simulink model "MATE_HDLsolver_myFirstCircuit"  (R2024b)
settings: Solver=FixedStepDiscrete  StartTime=0.0  StopTime=0.05  FixedStep=Ts  MaxStep=100e-6  RelTol=1e-4
PostLoadFcn:
  | Ts=1e-6; nb_sw=3; nb_lc=2;nb_r=1;nb_src=1; nb_out=3; rL=1.2;rC=100;L=1e-3; C=1e-5; LpejoSw=1e-6;h=Ts; MAX_INPUTS=16;
  | MAX_OUTPUTS=16;
  | MAX_SWITCHES=8;
  | MAX_INPUTS=16;
InitFcn:
  | Ts=1e-6; nb_sw=3; nb_lc=2;nb_r=1;nb_src=1; nb_out=3; rL=1.2;rC=100;L=1e-3; C=1e-5; LpejoSw=1e-6;h=Ts; MAX_INPUTS=16;
  | MAX_OUTPUTS=16;
  | MAX_SWITCHES=8;
  | MAX_INPUTS=16;
undefined symbols (not defined in the file or in its folder): MATE_SOC
libraries: fl_lib x31, nesl_utility x13, simetranss x5, simulink x2, ee_lib x2, eeGeneralControl x2
Description:
  | Copyright 2008-2010 The MathWorks, Inc.
settings Model: ARTEMISmethode_block_infos=$$__separator__$$  Creator=Kyle Diller
settings SolverCC: AlgebraicLoopSolver=TrustRegion
settings DataIOCC: SaveFormat=Array  SignalLoggingSaveFormat=ModelDataLogs  ReturnWorkspaceOutputs=off  SignalLoggingName=sigsOut
settings OptimizationCC: BlockReduction=off  BooleanDataType=off  ConditionallyExecuteInputs=off  OptimizeBlockIOStorage=off  BufferReuse=off  GlobalBufferReuse=off  ExpressionFolding=off  ExpressionDepthLimit=2147483647  LocalBlockOutputs=off  InitFltsAndDblsToZero=on  LifeSpan=inf
settings DebuggingCC: SaveWithParameterizedLinksMsg=none  UnderspecifiedInitializationDetection=Classic  MergeDetectMultiDrivingBlocksExec=none  CheckExecutionContextPreStartOutputMsg=on  SignalResolutionControl=TryResolveAllWithWarning  MultiTaskDSMMsg=warning  MultiTaskCondExecSysMsg=none  SigSpecEnsureSampleTimeMsg=none  FcnCallInpInsideContextMsg=warning  UnconnectedInputMsg=warning  UnconnectedOutputMsg=warning  UnconnectedLineMsg=warning  AllowSymbolicDim=off  StateNameClashWarn=warning  SFUnexpectedBacktrackingDiag=warning  SFNoUnconditionalDefaultTransitionDiag=warning  SFExecutionAtInitializationDiag=none  ArithmeticOperatorsInVariantConditions=warning
settings HardwareCC: ProdBitPerPointer=32  ProdBitPerSizeT=32  ProdBitPerPtrDiffT=32  ProdLargestAtomicFloat=None  ProdIntDivRoundTo=Undefined  ProdEndianess=Unspecified  ProdWordSize=32  ProdHWDeviceType=Specified  TargetUnknown=on
settings ModelReferenceCC: EnableRefExpFcnMdlSchedulingChecks=on  PropagateSignalLabelsOutOfModel=off
settings SFSimCC: SimUseLocalCustomCode=off  CustomCodeUndefinedFunction=UseInterfaceOnly
settings RTWCC: RTWUseLocalCustomCode=off  GPUComputeCapability=3.5
settings CodeAppCC: StateflowObjectComments=on
settings GRTTargetCC: TargetFcnLib=ansi_tfl_tmw.mat  TargetLangStandard=C89/C90 (ANSI)  CombineOutputUpdateFcns=off  GRTInterface=on
settings ConfigComp: CovMetricSettings=dw  CovSaveCumulativeToWorkspaceVar=on  CovSaveSingleToWorkspaceVar=on  CovExternalEMLEnable=off
settings SimscapeCC: SimscapeNormalizeSystem=off

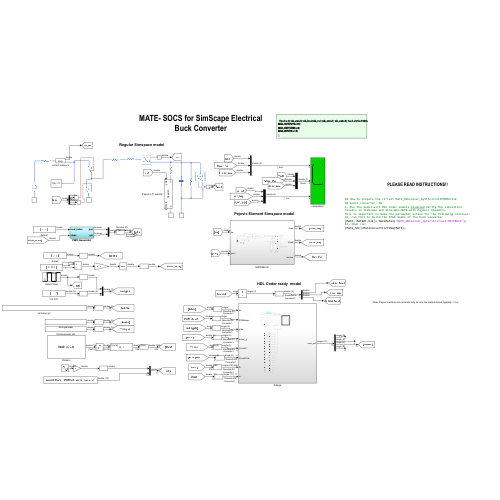
[thumbnail: Simulink's stored preview of the top-level diagram]
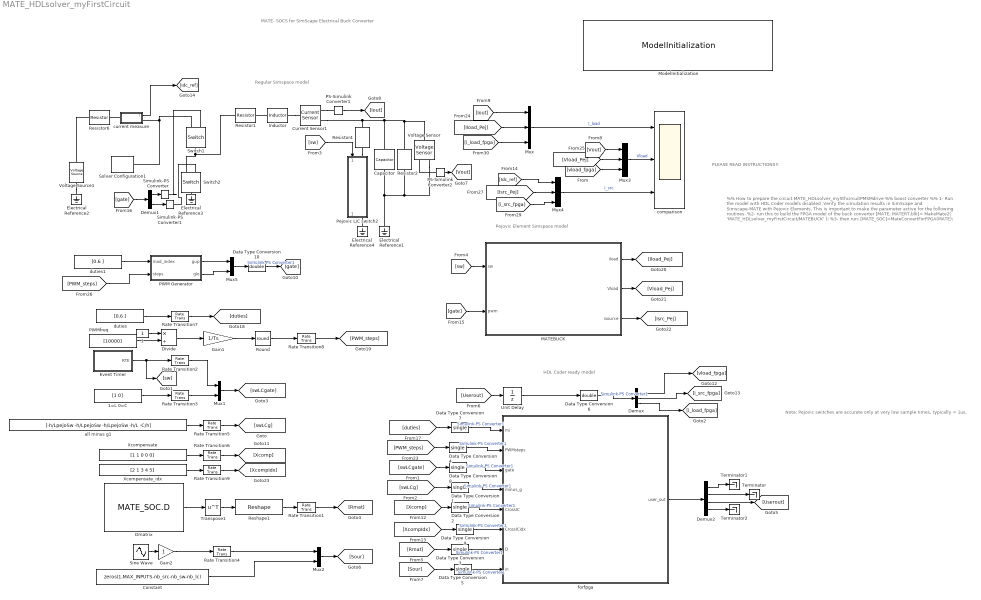
== system MATE_HDLsolver_myFirstCircuit ==
  note: Regular Simspace model
  note: Note: Pejovic switches are accurate only at very low sample times, typically < 1us,
  note: MATE- SOCS for SimScape Electrical
      | Buck Converter
  note: Pejovic Element Simspace model
  note: PLEASE READ INSTRUCTIONS!!
  note: %% How to prepare the circuit MATE_HDLsolver_my5thcircuitPMSMdrive
      | %% boost converter %%
      | 1- Run the model with HDL Coder models disabled .Verify the simulation results in SimScape and Simscape-MATE with Pejovic Elements.
      | This is important to make the parameter active for the following routines.
      | %2- run this to build the FPGA model of the buck converter
      | [MATE, MATERT,blk]= MakeMate2( 'MATE_HDLsolver_myFirstCircuit/MATEBUCK' );
      | %3- then run:
      | [MATE_SOC]=MateConvertForFPGA(MATE);
  note: HDL Coder ready model
  " Event Timer" : Subsystem  Tag=RTEcontrol_s38shd7k88  LoadFcn=|  mask(Timer){is=0 (off), t=[0.01 0.02 0.03 0.04 ], Tmax=0.07, Ts=Ts}
      | xx=get_param(gcb,'linkstatus');      
      | if isequal(xx,'inactive')            
      | set_param(gcb,'linkstatus','restore')
      | end
      mask prompts: is "Initial state"; t "Transition times (s):"; Tmax "Repeat period (s)"; Ts "Sample time (s)"
      mask help: This block generates a Simulink control signal changing at specified transition times.
      mask init:
      | iss=get_param(gcb,'is');
      | if isequal(iss,'0 (off)')
      |     sw(1)=0;
      |     sw(2)=0;
      | else
      |     sw(1)=1;
      |     sw(2)=1;
      | end
      | st(1)=0;
      | st(2)=t(1);
      | 
      | if t(1)==0,
      |    h=errordlg(' The first time specified must be greater than 0 ' , 'Parameter error');
      | end
      | 
      | i=3;
      | tog=0;
      | ptr=2;
      | while length(sw)<=2*length(t)
      |     if tog==0
      |         st=[st st(end)+Ts];
      |         sw=[sw 1-sw(end)];
      |         tog=1;
      |     else
      |         st=[st t(ptr)];
      |         sw=[sw sw(end)];
      |         ptr=ptr+1;
      |         tog=0;
      |     end
      | 
      | end
      |  %st=[st Tmax-Ts Tmax+Ts]
      | % sw=[sw sw(end) sw(1)]
      mask TypeOptions is: 0 (off) | 1 (on)
      mask Display:
      | %plot(0,0,100,100,[70,40,40,20,20,13],[30,30,70,70,30,30]);
      | plot( st(1:end-1), sw(1:end-1) );
  1 : Constant
  1=L 0=C : Constant  Value=[1 0]
  Capacitor : fl_lib/Electrical/Electrical Elements/Capacitor  c=C F  r=0 Ohm  g=0 1/Ohm  i_specify=off  i_priority=None  i=0 A  i_nominal_specify=off  i_nominal_value=1  i_nominal_unit=A  v_specify=off  v_priority=None  v=0 V  v_nominal_specify=off  v_nominal_value=1  v_nominal_unit=V  vc_specify=off  vc_priority=High  vc=0 V  vc_nominal_specify=off  vc_nominal_value=1  vc_nominal_unit=V
  Constant : Constant  Value=zeros(1,MAX_INPUTS-nb_src-nb_sw-nb_lc)
  Current Sensor1 : fl_lib/Electrical/Electrical Sensors/Current Sensor
  Data Type Conversion{1..5,7..9} (8 alike) : DataTypeConversion  OutDataTypeStr=single  RndMeth=Nearest  SaturateOnIntegerOverflow=off
  Data Type Conversion10 : DataTypeConversion  OutDataTypeStr=double  RndMeth=Nearest  SaturateOnIntegerOverflow=off
  Data Type Conversion6 : DataTypeConversion  OutDataTypeStr=double  RndMeth=Nearest  SaturateOnIntegerOverflow=off
  Demux : Demux  Outputs=3
  Demux1 : Demux  Outputs=2
  Demux2 : Demux  Outputs=[nb_sw nb_lc nb_out MAX_OUTPUTS-nb_out-nb_sw-nb_lc]
  Divide : Product  Inputs=*/
  Dmatrix : Constant  Value=MATE_SOC.D
  Electrical Reference{1..4} (4 alike) : fl_lib/Electrical/Electrical Elements/Electrical Reference
  Gain1 : Gain  Gain=1/Ts
  Gain2 : Gain
  Inductor : fl_lib/Electrical/Electrical Elements/Inductor  l=L H  r=0 Ohm  g=1e-9 1/Ohm  i_specify=off  i_priority=None  i=0 A  i_nominal_specify=off  i_nominal_value=1  i_nominal_unit=A  v_specify=off  v_priority=None  v=0 V  v_nominal_specify=off  v_nominal_value=1  v_nominal_unit=V  i_L_specify=off  i_L_priority=High  i_L=0 A  i_L_nominal_specify=off  i_L_nominal_value=1  i_L_nominal_unit=A
  MATEBUCK : Subsystem
  ModelInitialization : simetranss/Usefulls/ModelInitialization  InitFcnX=|  prel=off  posl=on  inif=on  strf=off
      | Ts=1e-6; nb_sw=3; nb_lc=2;nb_r=1;nb_src=1; nb_out=3; rL=1.2;rC=100;L=1e-3; C=1e-5; LpejoSw=1e-6;h=Ts; MAX_INPUTS=16;
      | MAX_OUTPUTS=16;
      | MAX_SWITCHES=8;
      | MAX_INPUTS=16;
  Mux : Mux  Inputs=3
  Mux1 : Mux  Inputs=2
  Mux2 : Mux  Inputs=2
  Mux3 : Mux  Inputs=3
  Mux4 : Mux  Inputs=3
  Mux5 : Mux  Inputs=2
  PS-Simulink Converter1 : nesl_utility/PS-Simulink Converter  PhysicalDomain=network_engine_domain  SubClassName=ps_output  LeftPortType=input  RightPortType=output  PseudoPeriodic=off  Frequencies=[]  VectorFormat=inherit  Unit=inherit  AffineConversion=off
  PS-Simulink Converter2 : nesl_utility/PS-Simulink Converter  PhysicalDomain=network_engine_domain  SubClassName=ps_output  LeftPortType=input  RightPortType=output  PseudoPeriodic=off  Frequencies=[]  VectorFormat=inherit  Unit=inherit  AffineConversion=off
  PWM Generator : Subsystem  Tag=RTEcontrol_s38shd7k88
  PWMfreq : Constant  Value=[10000]
  Pejovic L/C switch2 : Subsystem  AncestorBlock=simetranss/FPGA/Pejovic L//C switch  mask(Pejovic Switch){Lon=LpejoSw, Ts=Ts}
      mask prompts: Lon "Selected equivalent ON inductance (H)"; Ts "Sample Time (s)"
      mask help:
      | Pejovic switch model in SimScape
      |
      | Implements a single phase switch model using the Pejovic constant admittance method.
      | The user only has to select the equivalent ON-state inductance of the model, the corresponding Capacitance is computed internally.
      |
      | In the Pejovic model, Ts/Lon=Coff/Ts (Backward Euler) resulting in a constant admittance for the DAE solver.
      |
      | Input signals;
      |
      | gate: the switch gate value (1 for ON , 0 for OFF)
      mask init:
      | Coff=Ts*Ts/Lon;
      | Rsw=Lon/Ts;
      | 
      | if Ts>2e-6
      |     warndlg(['Sample Time of ' num2str(Ts) ' s. may be somehow large for the Pejovic switch to be accurate. Sample time below 2 us are recommended.'])
      | end
      mask Display: disp(['Pswitch'])
  Rate Transition{1..9} (9 alike) : RateTransition  OutPortSampleTime=1e-06
  Reshape1 : Reshape
  Resistor1 : fl_lib/Electrical/Electrical Elements/Resistor  R=rL Ohm  i_specify=off  i_priority=None  i=0 A  i_nominal_specify=off  i_nominal_value=1  i_nominal_unit=A  v_specify=off  v_priority=None  v=0 V  v_nominal_specify=off  v_nominal_value=1  v_nominal_unit=V
  Resistor2 : fl_lib/Electrical/Electrical Elements/Resistor  R=rC Ohm  i_specify=off  i_priority=None  i=0 A  i_nominal_specify=off  i_nominal_value=1  i_nominal_unit=A  v_specify=off  v_priority=None  v=0 V  v_nominal_specify=off  v_nominal_value=1  v_nominal_unit=V
  Resistor4 : fl_lib/Electrical/Electrical Elements/Resistor  R=rC Ohm  i_specify=off  i_priority=None  i=0 A  i_nominal_specify=off  i_nominal_value=1  i_nominal_unit=A  v_specify=off  v_priority=None  v=0 V  v_nominal_specify=off  v_nominal_value=1  v_nominal_unit=V
  Resistor6 : fl_lib/Electrical/Electrical Elements/Resistor  R=0.01 Ohm  i_specify=off  i_priority=None  i=0 A  i_nominal_specify=off  i_nominal_value=1  i_nominal_unit=A  v_specify=off  v_priority=None  v=0 V  v_nominal_specify=off  v_nominal_value=1  v_nominal_unit=V
  Round : Rounding  Operator=round
  Simulink-PS Converter : nesl_utility/Simulink-PS Converter  PhysicalDomain=network_engine_domain  SubClassName=ps_input  LeftPortType=input  RightPortType=output  PseudoPeriodic=off  Frequencies=[]  NoiseDistribution=none  NoiseParameters=[]  Unit=1  AffineConversion=off  FilteringAndDerivatives=provide  SimscapeFilterOrder=1  InputFilterTimeConstant=0.001  UdotUserProvided=0
  Simulink-PS Converter1 : nesl_utility/Simulink-PS Converter  PhysicalDomain=network_engine_domain  SubClassName=ps_input  LeftPortType=input  RightPortType=output  PseudoPeriodic=off  Frequencies=[]  NoiseDistribution=none  NoiseParameters=[]  Unit=1  AffineConversion=off  FilteringAndDerivatives=provide  SimscapeFilterOrder=1  InputFilterTimeConstant=0.001  UdotUserProvided=0
  Sine Wave : Sin  Amplitude=0  Bias=100  Frequency=0  SampleTime=0
  Solver Configuration1 : nesl_utility/Solver Configuration  PhysicalDomain=network_engine_domain  SubClassName=solver  LeftPortType=input  RightPortType=generic  Tones=[]  Harmonics=[]  SimulateNoise=off  Profile=off  UseLocalSampling=off  EnableSwitchedLinearOptims=on  FrequencyDomain=off  UseCCode=off  RelTol=0.001  AbsTol=0.001  MinStep=1e-09  ToWorkspace=off  RevertToSquareIcSolve=off  NumHomotopyIterations=100  PhasorMode=off  PhasorModeNumHarmonics=1  ConsistencySolver=NEWTON_XTOL_AFTER_FTOL  IndexReductionMethod=DerivativeReplacement  DoDC=off  ResidualTolerance=1e-09  ConsistencyTolSource=GLOBAL  ConsistencyAbsTol=0.001  ConsistencyRelTol=0.001  ConsistencyTolFactor=0.001  UseLocalSolver=on  LocalSolverChoice=NE_BACKWARD_EULER_ADVANCER  ResolveIndetEquations=on  FunctionEvalNumThread=1  LocalSolverSampleTime=Ts  DoFixedCost=on  MaxNonlinIter=1  MaxModeIter=2  ComputeImpulses=off  ImpulseIterations=2  LinearAlgebra=auto  LinearAlgebraNumThread=0  EquationFormulation=NE_TIME_EF  DelaysMemoryBudget=1024  AutomaticFiltering=on  FilteringTimeConstant=0.001  PartitionStorageMethod=AS_NEEDED  PartitionMemoryBudget=1024  PartitionMethod=ROBUST  MultibodyUseLocalSolver=off  MultibodyLocalSolverChoice=ODE1  MultibodyLocalSolverSampleTime=0.001
  Switch1 : fl_lib/Electrical/Electrical Elements/Switch  R_closed=0.001 Ohm  G_open=1e-8 1/Ohm  Threshold=0.5  i_specify=off  i_priority=None  i=0 A  i_nominal_specify=off  i_nominal_value=1  i_nominal_unit=A  v_specify=off  v_priority=None  v=0 V  v_nominal_specify=off  v_nominal_value=1  v_nominal_unit=V
  Switch2 : fl_lib/Electrical/Electrical Elements/Switch  R_closed=0.001 Ohm  G_open=1e-8 1/Ohm  Threshold=0.5  i_specify=off  i_priority=None  i=0 A  i_nominal_specify=off  i_nominal_value=1  i_nominal_unit=A  v_specify=off  v_priority=None  v=0 V  v_nominal_specify=off  v_nominal_value=1  v_nominal_unit=V
  Terminator : Terminator
  Terminator1 : Terminator
  Terminator2 : Terminator
  Transpose1 : Math  Operator=transpose
  Unit Delay : UnitDelay  SampleTime=-1  HasFrameUpgradeWarning=on
  Voltage Sensor : fl_lib/Electrical/Electrical Sensors/Voltage Sensor
  Voltage Source1 : ee_lib/Sources/Voltage Source  dc_voltage=100 V  ac_voltage=0 V  ac_shift=0 rad  ac_frequency=60 Hz  noise_mode=ee.enum.sources.noise.Disabled  PSD=0 V^2/Hz  sample_time=1e-3 s  repeatability=ee.enum.sources.repeatability.NotRepeatable  user_seed=0  auto_seed=1196140742  i_specify=off  i_priority=None  i=0 A  i_nominal_specify=off  i_nominal_value=1  i_nominal_unit=A  v_specify=off  v_priority=None  v=0 V  v_nominal_specify=off  v_nominal_value=1  v_nominal_unit=V
  Xcompensate : Constant  Value=[1 1 0 0 0]
  Xcompensate_idx : Constant  Value=[2 1 3 4 5]
  all minus g1 : Constant  Value=[-h/LpejoSw -h/LpejoSw -h/LpejoSw -h/L -C/h]
  comparison : Scope  NumInputPorts=3
  current measure : Subsystem
      mask Display: disp('amp')
  duties : Constant  Value=[0.6 ]
  duties1 : Constant  Value=[0.6 ]
  forfpga : Subsystem
  wires:
  [sw] -> Pejovic L/C switch2/1(gate)
  Mux/1 -> comparison/1  "I_load"
  Dmatrix/1 -> Transpose1/1
  " Event Timer"/1(RTE) -> [sw], Rate Transition2/1
  Rate Transition2/1 -> Mux1/1
  Sine Wave/1 -> Gain2/1
  Unit Delay/1 -> Data Type Conversion6/1
  1=L 0=C/1 -> Rate Transition3/1
  Rate Transition3/1 -> Mux1/2
  Mux3/1 -> comparison/2  "Vload"
  [Vout] -> Mux3/1
  [sw] -> MATEBUCK/1(sw)
  Mux1/1 -> [swLCgate]
  all minus g1/1 -> Rate Transition5/1
  Rate Transition5/1 -> [swLCg]
  Gain2/1 -> Rate Transition4/1
  Rate Transition1/1 -> [Rmat]
  [Userout] -> Unit Delay/1
  Rate Transition6/1 -> [Xcomp]
  Xcompensate/1 -> Rate Transition6/1
  [swLCgate] -> Data Type Conversion8/1
  [swLCg] -> Data Type Conversion1/1
  [Xcomp] -> Data Type Conversion2/1
  [Rmat] -> Data Type Conversion3/1
  [Sour] -> Data Type Conversion5/1
  Data Type Conversion8/1 -> forfpga/3(gate)  "Simulink-PS Converter1"
  Data Type Conversion1/1 -> forfpga/4(minus_g)  "Simulink-PS Converter1"
  Data Type Conversion2/1 -> forfpga/5(CrossIC)  "Simulink-PS Converter1"
  Data Type Conversion3/1 -> forfpga/7(D)  "Simulink-PS Converter1"
  Data Type Conversion5/1 -> forfpga/8(in)  "Simulink-PS Converter1"
  Demux/1 -> [vload_fpga]
  Demux/2 -> [i_src_fpga]
  [vload_fpga] -> Mux3/3
  Data Type Conversion6/1 -> Demux/1  "Simulink-PS Converter1"
  [gate] -> MATEBUCK/2(pwm)
  Demux1/2 -> Simulink-PS Converter1/1
  Demux1/1 -> Simulink-PS Converter/1
  [gate] -> Demux1/1
  current measure/1(i) -> [Idc_ref]
  duties/1 -> Rate Transition7/1
  Rate Transition7/1 -> [duties]
  Data Type Conversion7/1 -> forfpga/1(mi)  "Simulink-PS Converter1"
  [duties] -> Data Type Conversion7/1
  Mux2/1 -> [Sour]
  Rate Transition4/1 -> Mux2/1
  Constant/1 -> Mux2/2
  Data Type Conversion4/1 -> forfpga/2(PWMsteps)  "Simulink-PS Converter1"
  Rate Transition8/1 -> [PWM_steps]
  Divide/1 -> Gain1/1
  Gain1/1 -> Round/1
  [PWM_steps] -> Data Type Conversion4/1
  forfpga/1(user_out) -> Demux2/1
  Demux2/2 -> Terminator/1
  MATEBUCK/1(iload) -> [Iload_Pej]
  MATEBUCK/2(Vload) -> [Vload_Pej]
  MATEBUCK/3(isource) -> [Isrc_Pej]
  [Iload_Pej] -> Mux/2
  [i_load_fpga] -> Mux/3
  [Vload_Pej] -> Mux3/2
  Mux4/1 -> comparison/3  "I_src"
  [Idc_ref] -> Mux4/1
  [Isrc_Pej] -> Mux4/2
  Demux2/3 -> [Userout]
  Demux2/1 -> Terminator1/1
  Demux2/4 -> Terminator2/1
  PWMfreq/1 -> Divide/2
  1/1 -> Divide/1
  Demux/3 -> [i_load_fpga]
  [i_src_fpga] -> Mux4/3
  Xcompensate_idx/1 -> Rate Transition9/1
  Rate Transition9/1 -> [XcompIdx]
  [XcompIdx] -> Data Type Conversion9/1
  Data Type Conversion9/1 -> forfpga/6(CrossICidx)  "Simulink-PS Converter1"
  Round/1 -> Rate Transition8/1
  duties1/1 -> PWM Generator/1(mod_index)
  [PWM_steps] -> PWM Generator/2(steps)
  PWM Generator/2(glo) -> Mux5/2
  PWM Generator/1(gup) -> Mux5/1
  Mux5/1 -> Data Type Conversion10/1
  Data Type Conversion10/1 -> [gate]  "Simulink-PS Converter1"
  PS-Simulink Converter2/1 -> [Vout]
  PS-Simulink Converter1/1 -> [Iout]
  [Iout] -> Mux/1
  Transpose1/1 -> Reshape1/1
  Reshape1/1 -> Rate Transition1/1
  connections:
  Switch2/RConn2 -- Resistor1/LConn1 -- Switch1/LConn1
  Switch1/RConn2 -- current measure/RConn1 -- Solver Configuration1/RConn1
  Current Sensor1/RConn1 -- PS-Simulink Converter1/LConn1
  Inductor/LConn1 -- Resistor1/RConn1
  Inductor/RConn1 -- Current Sensor1/LConn1
  Current Sensor1/RConn2 -- Resistor4/LConn1 -- Voltage Sensor/LConn1 -- Resistor2/LConn1 -- Capacitor/LConn1
  Voltage Sensor/RConn2 -- Resistor2/RConn1 -- Capacitor/RConn1 -- Electrical Reference1/LConn1
  Voltage Source1/LConn1 -- Resistor6/LConn1
  Voltage Source1/RConn1 -- Electrical Reference2/LConn1
  Simulink-PS Converter1/RConn1 -- Switch2/RConn1
  Simulink-PS Converter/RConn1 -- Switch1/RConn1
  Electrical Reference3/LConn1 -- Switch2/LConn1
  current measure/LConn1 -- Resistor6/RConn1
  Electrical Reference4/LConn1 -- Pejovic L/C switch2/RConn1
  Resistor4/RConn1 -- Pejovic L/C switch2/LConn1
  PS-Simulink Converter2/LConn1 -- Voltage Sensor/RConn1

== system MATE_HDLsolver_myFirstCircuit/ Event Timer ==
  Repeating Sequence : simulink/Sources/Repeating Sequence  rep_seq_t=st  rep_seq_y=sw
  Repeating Sequence1 : simulink/Sources/Repeating Sequence  Commented=on  rep_seq_t="[0    0.2000    0.2001    0.4000    0.4001    0.6000    2.0000]"  rep_seq_y=|
      | [     1     1     0     0     1     1     1
      | ]
  RTE : Outport  VectorParamsAs1DForOutWhenUnconnected=off
  wires:
  Repeating Sequence/1 -> RTE/1

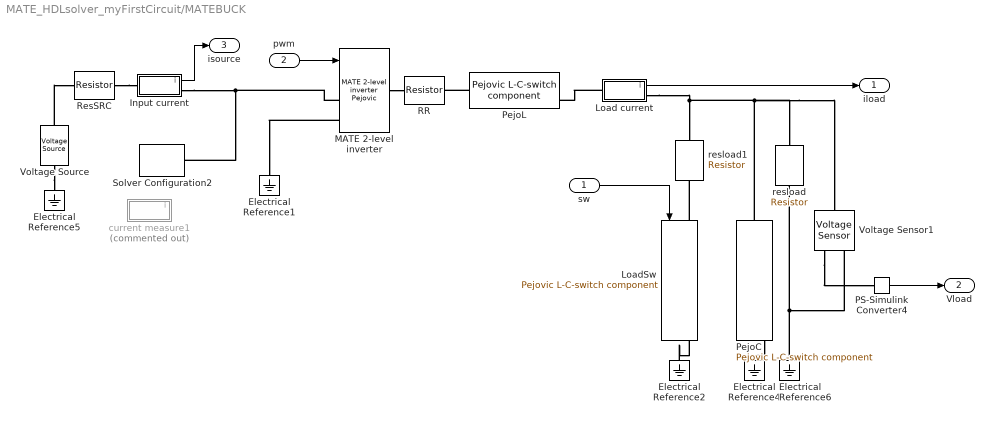
== system MATE_HDLsolver_myFirstCircuit/MATEBUCK ==
  sw : Inport
  pwm : Inport  Port=2
  Electrical Reference{1..2,4..6} (5 alike) : fl_lib/Electrical/Electrical Elements/Electrical Reference
  Input current : Subsystem
  Load current : Subsystem
  LoadSw : simetranss/FPGA/Pejovic L-C-switch component  typ=Switch  Lon=LpejoSw  L=L  C=C  otherSW='coming soon'  Ts=Ts  pcbp=off
  MATE 2-level inverter : simetranss/FPGA/MATE 2-level inverter Pejovic  Lon=1e-6  Ts=Ts
  PS-Simulink Converter4 : nesl_utility/PS-Simulink Converter  PhysicalDomain=network_engine_domain  SubClassName=ps_output  LeftPortType=input  RightPortType=output  PseudoPeriodic=off  Frequencies=[]  VectorFormat=inherit  Unit=inherit  AffineConversion=off
  PejoC : simetranss/FPGA/Pejovic L-C-switch component  typ=Capacitor  Lon=LpejoSw  L=L  C=C  otherSW='coming soon'  Ts=Ts  pcbp=off
  PejoL : simetranss/FPGA/Pejovic L-C-switch component  typ=Inductor  Lon=LpejoSw  L=L  C=C  otherSW='coming soon'  Ts=Ts  pcbp=off
  RR : fl_lib/Electrical/Electrical Elements/Resistor  R=rL Ohm  i_specify=off  i_priority=None  i=0 A  i_nominal_specify=off  i_nominal_value=1  i_nominal_unit=A  v_specify=off  v_priority=None  v=0 V  v_nominal_specify=off  v_nominal_value=1  v_nominal_unit=V
  ResSRC : fl_lib/Electrical/Electrical Elements/Resistor  R=0.01 Ohm  i_specify=off  i_priority=None  i=0 A  i_nominal_specify=off  i_nominal_value=1  i_nominal_unit=A  v_specify=off  v_priority=None  v=0 V  v_nominal_specify=off  v_nominal_value=1  v_nominal_unit=V
  Solver Configuration2 : nesl_utility/Solver Configuration  PhysicalDomain=network_engine_domain  SubClassName=solver  LeftPortType=input  RightPortType=generic  Tones=[]  Harmonics=[]  SimulateNoise=off  Profile=off  UseLocalSampling=off  EnableSwitchedLinearOptims=on  FrequencyDomain=off  UseCCode=off  RelTol=0.001  AbsTol=0.001  MinStep=1e-09  ToWorkspace=off  RevertToSquareIcSolve=off  NumHomotopyIterations=100  PhasorMode=off  PhasorModeNumHarmonics=1  ConsistencySolver=NEWTON_XTOL_AFTER_FTOL  IndexReductionMethod=DerivativeReplacement  DoDC=off  ResidualTolerance=1e-09  ConsistencyTolSource=GLOBAL  ConsistencyAbsTol=0.001  ConsistencyRelTol=0.001  ConsistencyTolFactor=0.001  UseLocalSolver=on  LocalSolverChoice=NE_BACKWARD_EULER_ADVANCER  ResolveIndetEquations=on  FunctionEvalNumThread=1  LocalSolverSampleTime=Ts  DoFixedCost=on  MaxNonlinIter=1  MaxModeIter=2  ComputeImpulses=off  ImpulseIterations=2  LinearAlgebra=auto  LinearAlgebraNumThread=0  EquationFormulation=NE_TIME_EF  DelaysMemoryBudget=1024  AutomaticFiltering=on  FilteringTimeConstant=0.001  PartitionStorageMethod=AS_NEEDED  PartitionMemoryBudget=1024  PartitionMethod=ROBUST  MultibodyUseLocalSolver=off  MultibodyLocalSolverChoice=ODE1  MultibodyLocalSolverSampleTime=0.001
  Voltage Sensor1 : fl_lib/Electrical/Electrical Sensors/Voltage Sensor
  Voltage Source : ee_lib/Sources/Voltage Source  dc_voltage=100 V  ac_voltage=0 V  ac_shift=0 rad  ac_frequency=60 Hz  noise_mode=ee.enum.sources.noise.Disabled  PSD=0 V^2/Hz  sample_time=1e-3 s  repeatability=ee.enum.sources.repeatability.NotRepeatable  user_seed=0  auto_seed=198304613  i_specify=off  i_priority=None  i=0 A  i_nominal_specify=off  i_nominal_value=1  i_nominal_unit=A  v_specify=off  v_priority=None  v=0 V  v_nominal_specify=off  v_nominal_value=1  v_nominal_unit=V
  current measure1 : Subsystem  Commented=on
      mask Display: disp('amp')
  resload : fl_lib/Electrical/Electrical Elements/Resistor  R=rC Ohm  i_specify=off  i_priority=None  i=0 A  i_nominal_specify=off  i_nominal_value=1  i_nominal_unit=A  v_specify=off  v_priority=None  v=0 V  v_nominal_specify=off  v_nominal_value=1  v_nominal_unit=V
  resload1 : fl_lib/Electrical/Electrical Elements/Resistor  R=rC Ohm  i_specify=off  i_priority=None  i=0 A  i_nominal_specify=off  i_nominal_value=1  i_nominal_unit=A  v_specify=off  v_priority=None  v=0 V  v_nominal_specify=off  v_nominal_value=1  v_nominal_unit=V
  iload : Outport
  Vload : Outport  Port=2
  isource : Outport  Port=3
  wires:
  PS-Simulink Converter4/1 -> Vload/1
  sw/1 -> LoadSw/1
  Load current/1(i) -> iload/1
  pwm/1 -> MATE 2-level inverter/1
  Input current/1(i) -> isource/1
  connections:
  Load current/LConn1 -- PejoL/RConn1
  Voltage Source/RConn1 -- Electrical Reference5/LConn1
  Voltage Source/LConn1 -- ResSRC/LConn1
  MATE 2-level inverter/RConn1 -- RR/LConn1
  PejoL/LConn1 -- RR/RConn1
  PejoC/RConn1 -- Electrical Reference4/LConn1
  Voltage Sensor1/RConn1 -- PS-Simulink Converter4/LConn1
  Electrical Reference6/LConn1 -- resload/RConn1 -- Voltage Sensor1/RConn2
  Input current/RConn1 -- MATE 2-level inverter/LConn1 -- Solver Configuration2/RConn1
  Voltage Sensor1/LConn1 -- resload/LConn1 -- Load current/RConn1 -- resload1/LConn1 -- PejoC/LConn1
  MATE 2-level inverter/LConn2 -- Electrical Reference1/LConn1
  LoadSw/LConn1 -- resload1/RConn1
  Electrical Reference2/LConn1 -- LoadSw/RConn1
  ResSRC/RConn1 -- Input current/LConn1

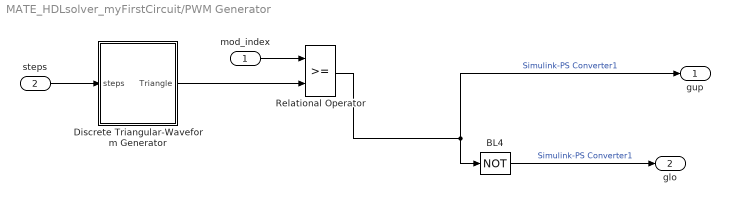
== system MATE_HDLsolver_myFirstCircuit/PWM Generator ==
  mod_index : Inport
  steps : Inport  Port=2
  BL4 : Logic  Operator=NOT  Inputs=1
  Discrete Triangular-Waveform Generator : Subsystem
  Relational Operator : RelationalOperator  OutDataTypeStr=boolean
  gup : Outport  VectorParamsAs1DForOutWhenUnconnected=off
  glo : Outport  Port=2  VectorParamsAs1DForOutWhenUnconnected=off
  wires:
  Discrete Triangular-Waveform Generator/1(Triangle) -> Relational Operator/2
  mod_index/1 -> Relational Operator/1
  steps/1 -> Discrete Triangular-Waveform Generator/1(steps)
  Relational Operator/1 -> gup/1, BL4/1  "Simulink-PS Converter1"
  BL4/1 -> glo/1  "Simulink-PS Converter1"

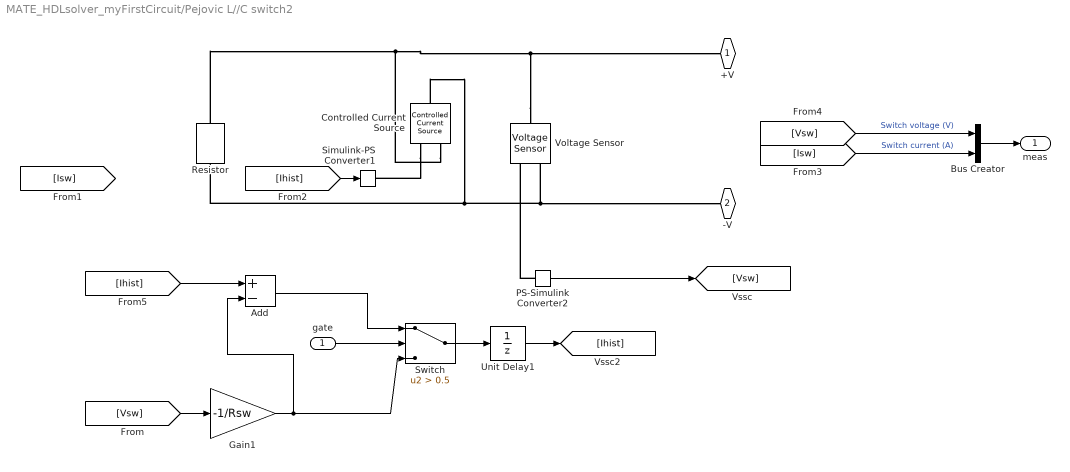
== system MATE_HDLsolver_myFirstCircuit/Pejovic L//C switch2 ==
  gate : Inport
  Add : Sum  Inputs=+-
  Bus Creator : BusCreator  Inputs=2
  Controlled Current Source : fl_lib/Electrical/Electrical Sources/Controlled Current Source
  Gain1 : Gain  Gain=-1/Rsw
  PS-Simulink Converter2 : nesl_utility/PS-Simulink Converter  PhysicalDomain=network_engine_domain  SubClassName=ps_output  LeftPortType=input  RightPortType=output  PseudoPeriodic=off  Frequencies=[]  VectorFormat=inherit  Unit=inherit  AffineConversion=off
  Resistor : fl_lib/Electrical/Electrical Elements/Resistor  R=Rsw Ohm  i_specify=off  i_priority=None  i=0 A  i_nominal_specify=off  i_nominal_value=1  i_nominal_unit=A  v_specify=off  v_priority=None  v=0 V  v_nominal_specify=off  v_nominal_value=1  v_nominal_unit=V
  Simulink-PS Converter1 : nesl_utility/Simulink-PS Converter  PhysicalDomain=network_engine_domain  SubClassName=ps_input  LeftPortType=input  RightPortType=output  PseudoPeriodic=off  Frequencies=[]  NoiseDistribution=none  NoiseParameters=[]  Unit=1  AffineConversion=off  FilteringAndDerivatives=provide  SimscapeFilterOrder=1  InputFilterTimeConstant=0.001  UdotUserProvided=0
  Switch : Switch  Criteria=u2 > Threshold  Threshold=0.5  SaturateOnIntegerOverflow=off  InputSameDT=off
  Unit Delay1 : UnitDelay  SampleTime=-1  HasFrameUpgradeWarning=on
  Voltage Sensor : fl_lib/Electrical/Electrical Sensors/Voltage Sensor
  +V : PMIOPort  Side=Left
  -V : PMIOPort  Port=2  Side=Right
  meas : Outport
  wires:
  Unit Delay1/1 -> [Ihist]
  Add/1 -> Switch/1
  Gain1/1 -> Add/2, Switch/3
  [Ihist] -> Add/1
  PS-Simulink Converter2/1 -> [Vsw]
  gate/1 -> Switch/2
  [Vsw] -> Gain1/1
  Switch/1 -> Unit Delay1/1
  [Ihist] -> Simulink-PS Converter1/1
  [Isw] -> Bus Creator/2  "Switch current (A)"
  [Vsw] -> Bus Creator/1  "Switch voltage (V)"
  Bus Creator/1 -> meas/1
  connections:
  Resistor/RConn1 -- Controlled Current Source/LConn1 -- Voltage Sensor/RConn2 -- -V/RConn1
  PS-Simulink Converter2/LConn1 -- Voltage Sensor/RConn1
  Controlled Current Source/RConn1 -- Simulink-PS Converter1/RConn1
  Voltage Sensor/LConn1 -- +V/RConn1 -- Controlled Current Source/RConn2 -- Resistor/LConn1

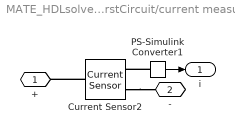
== system MATE_HDLsolver_myFirstCircuit/current measure ==
  Current Sensor2 : fl_lib/Electrical/Electrical Sensors/Current Sensor
  PS-Simulink Converter1 : nesl_utility/PS-Simulink Converter  PhysicalDomain=network_engine_domain  SubClassName=ps_output  LeftPortType=input  RightPortType=output  PseudoPeriodic=off  Frequencies=[]  VectorFormat=inherit  Unit=inherit  AffineConversion=off
  + : PMIOPort  Side=Left
  - : PMIOPort  Port=2  Side=Right
  i : Outport
  wires:
  PS-Simulink Converter1/1 -> i/1
  connections:
  PS-Simulink Converter1/LConn1 -- Current Sensor2/RConn1
  Current Sensor2/LConn1 -- +/RConn1
  Current Sensor2/RConn2 -- -/RConn1

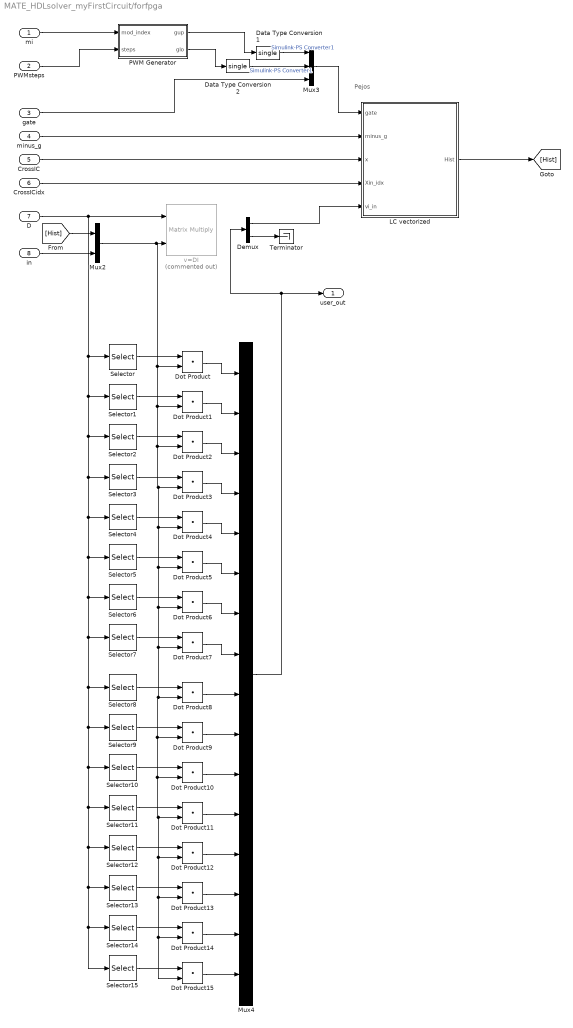
== system MATE_HDLsolver_myFirstCircuit/forfpga ==
  note: Pejos
  mi : Inport
  PWMsteps : Inport  Port=2
  gate : Inport  Port=3
  minus_g : Inport  Port=4
  CrossIC : Inport  Port=5
  CrossICidx : Inport  Port=6
  D : Inport  Port=7
  in : Inport  Port=8
  Data Type Conversion1 : DataTypeConversion  OutDataTypeStr=single  RndMeth=Nearest  SaturateOnIntegerOverflow=off
  Data Type Conversion2 : DataTypeConversion  OutDataTypeStr=single  RndMeth=Nearest  SaturateOnIntegerOverflow=off
  Demux : Demux  Outputs=[nb_sw+nb_lc -1]
  Dot Product{,1..15} (16 alike) : DotProduct  OutDataTypeStr=Inherit: Inherit via internal rule
  LC vectorized : Subsystem
  Mux2 : Mux  Inputs=2
  Mux3 : Mux  Inputs=3
  Mux4 : Mux  Inputs=16
  PWM Generator : Subsystem  Tag=RTEcontrol_s38shd7k88
  Selector : Selector  InputPortWidth=16*16  IndexOptions=Index vector (dialog)  Indices=[1:16]  OutputSizes=1
  Selector1 : Selector  InputPortWidth=16*16  IndexOptions=Index vector (dialog)  Indices=[1:16]+16*1  OutputSizes=1
  Selector10 : Selector  InputPortWidth=16*16  IndexOptions=Index vector (dialog)  Indices=[1:16]+16*10  OutputSizes=1
  Selector11 : Selector  InputPortWidth=16*16  IndexOptions=Index vector (dialog)  Indices=[1:16]+16*11  OutputSizes=1
  Selector12 : Selector  InputPortWidth=16*16  IndexOptions=Index vector (dialog)  Indices=[1:16]+16*12  OutputSizes=1
  Selector13 : Selector  InputPortWidth=16*16  IndexOptions=Index vector (dialog)  Indices=[1:16]+16*13  OutputSizes=1
  Selector14 : Selector  InputPortWidth=16*16  IndexOptions=Index vector (dialog)  Indices=[1:16]+16*14  OutputSizes=1
  Selector15 : Selector  InputPortWidth=16*16  IndexOptions=Index vector (dialog)  Indices=[1:16]+16*15  OutputSizes=1
  Selector2 : Selector  InputPortWidth=16*16  IndexOptions=Index vector (dialog)  Indices=[1:16]+16*2  OutputSizes=1
  Selector3 : Selector  InputPortWidth=16*16  IndexOptions=Index vector (dialog)  Indices=[1:16]+16*3  OutputSizes=1
  Selector4 : Selector  InputPortWidth=16*16  IndexOptions=Index vector (dialog)  Indices=[1:16]+16*4  OutputSizes=1
  Selector5 : Selector  InputPortWidth=16*16  IndexOptions=Index vector (dialog)  Indices=[1:16]+16*5  OutputSizes=1
  Selector6 : Selector  InputPortWidth=16*16  IndexOptions=Index vector (dialog)  Indices=[1:16]+16*6  OutputSizes=1
  Selector7 : Selector  InputPortWidth=16*16  IndexOptions=Index vector (dialog)  Indices=[1:16]+16*7  OutputSizes=1
  Selector8 : Selector  InputPortWidth=16*16  IndexOptions=Index vector (dialog)  Indices=[1:16]+16*8  OutputSizes=1
  Selector9 : Selector  InputPortWidth=16*16  IndexOptions=Index vector (dialog)  Indices=[1:16]+16*9  OutputSizes=1
  Terminator : Terminator
  v=DI : Product  Commented=on  Multiplication=Matrix(*)
  user_out : Outport
  wires:
  in/1 -> Mux2/2
  LC vectorized/1(Hist) -> [Hist]
  minus_g/1 -> LC vectorized/2(minus_g)
  CrossIC/1 -> LC vectorized/3(x)
  Demux/1 -> LC vectorized/5(vi_in)
  mi/1 -> PWM Generator/1(mod_index)
  PWM Generator/1(gup) -> Data Type Conversion1/1
  Mux3/1 -> LC vectorized/1(gate)
  PWMsteps/1 -> PWM Generator/2(steps)
  gate/1 -> Mux3/3
  PWM Generator/2(glo) -> Data Type Conversion2/1
  Demux/2 -> Terminator/1
  [Hist] -> Mux2/1
  Data Type Conversion1/1 -> Mux3/1  "Simulink-PS Converter1"
  Data Type Conversion2/1 -> Mux3/2  "Simulink-PS Converter1"
  CrossICidx/1 -> LC vectorized/4(Xin_idx)
  Selector7/1 -> Dot Product7/1
  Dot Product10/1 -> Mux4/11
  Dot Product9/1 -> Mux4/10
  Dot Product13/1 -> Mux4/14
  Dot Product8/1 -> Mux4/9
  Dot Product11/1 -> Mux4/12
  Dot Product15/1 -> Mux4/16
  Dot Product6/1 -> Mux4/7
  Dot Product/1 -> Mux4/1
  Selector3/1 -> Dot Product3/1
  Dot Product5/1 -> Mux4/6
  Selector2/1 -> Dot Product2/1
  Dot Product1/1 -> Mux4/2
  Dot Product2/1 -> Mux4/3
  Mux4/1 -> Demux/1, user_out/1
  Dot Product7/1 -> Mux4/8
  Selector8/1 -> Dot Product8/1
  Selector10/1 -> Dot Product10/1
  Selector15/1 -> Dot Product15/1
  Selector12/1 -> Dot Product12/1
  Selector11/1 -> Dot Product11/1
  Dot Product12/1 -> Mux4/13
  Selector13/1 -> Dot Product13/1
  Selector4/1 -> Dot Product4/1
  Selector/1 -> Dot Product/1
  Selector6/1 -> Dot Product6/1
  Selector9/1 -> Dot Product9/1
  D/1 -> v=DI/1, Selector1/1, Selector2/1, Selector3/1, Selector4/1, Selector5/1, Selector8/1, Selector14/1, Selector15/1, Selector13/1, Selector12/1, Selector11/1, Selector10/1, Selector9/1, Selector7/1, Selector6/1, Selector/1
  Dot Product14/1 -> Mux4/15
  Selector14/1 -> Dot Product14/1
  Selector1/1 -> Dot Product1/1
  Mux2/1 -> Dot Product9/2, Dot Product10/2, Dot Product11/2, Dot Product12/2, Dot Product13/2, Dot Product14/2, Dot Product15/2, Dot Product8/2, Dot Product7/2, Dot Product6/2, Dot Product5/2, Dot Product4/2, Dot Product3/2, Dot Product2/2, Dot Product1/2, Dot Product/2, v=DI/2
  Dot Product3/1 -> Mux4/4
  Selector5/1 -> Dot Product5/1
  Dot Product4/1 -> Mux4/5

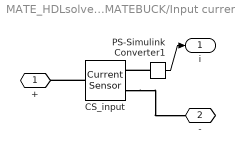
== system MATE_HDLsolver_myFirstCircuit/MATEBUCK/Input current ==
  CS_input : fl_lib/Electrical/Electrical Sensors/Current Sensor
  PS-Simulink Converter1 : nesl_utility/PS-Simulink Converter  PhysicalDomain=network_engine_domain  SubClassName=ps_output  LeftPortType=input  RightPortType=output  PseudoPeriodic=off  Frequencies=[]  VectorFormat=inherit  Unit=inherit  AffineConversion=off
  + : PMIOPort  Side=Left
  - : PMIOPort  Port=2  Side=Right
  i : Outport
  wires:
  PS-Simulink Converter1/1 -> i/1
  connections:
  PS-Simulink Converter1/LConn1 -- CS_input/RConn1
  CS_input/LConn1 -- +/RConn1
  CS_input/RConn2 -- -/RConn1

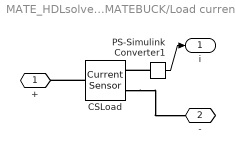
== system MATE_HDLsolver_myFirstCircuit/MATEBUCK/Load current ==
  CSLoad : fl_lib/Electrical/Electrical Sensors/Current Sensor
  PS-Simulink Converter1 : nesl_utility/PS-Simulink Converter  PhysicalDomain=network_engine_domain  SubClassName=ps_output  LeftPortType=input  RightPortType=output  PseudoPeriodic=off  Frequencies=[]  VectorFormat=inherit  Unit=inherit  AffineConversion=off
  + : PMIOPort  Side=Left
  - : PMIOPort  Port=2  Side=Right
  i : Outport
  wires:
  PS-Simulink Converter1/1 -> i/1
  connections:
  CSLoad/RConn2 -- -/RConn1
  CSLoad/LConn1 -- +/RConn1
  PS-Simulink Converter1/LConn1 -- CSLoad/RConn1

== system MATE_HDLsolver_myFirstCircuit/MATEBUCK/current measure1 ==
  Current Sensor2 : fl_lib/Electrical/Electrical Sensors/Current Sensor
  PS-Simulink Converter1 : nesl_utility/PS-Simulink Converter  PhysicalDomain=network_engine_domain  SubClassName=ps_output  LeftPortType=input  RightPortType=output  PseudoPeriodic=off  Frequencies=[]  VectorFormat=inherit  Unit=inherit  AffineConversion=off
  + : PMIOPort  Side=Left
  - : PMIOPort  Port=2  Side=Right
  i : Outport
  wires:
  PS-Simulink Converter1/1 -> i/1
  connections:
  Current Sensor2/RConn2 -- -/RConn1
  Current Sensor2/LConn1 -- +/RConn1
  PS-Simulink Converter1/LConn1 -- Current Sensor2/RConn1

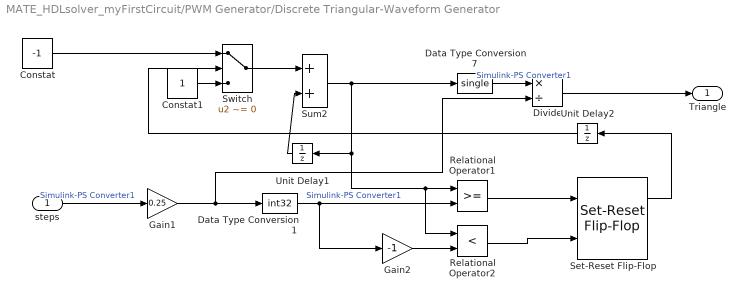
== system MATE_HDLsolver_myFirstCircuit/PWM Generator/Discrete Triangular-Waveform Generator ==
  steps : Inport
  Constat : Constant  Value=-1  OutDataTypeStr=int32
  Constat1 : Constant  OutDataTypeStr=int32
  Data Type Conversion1 : DataTypeConversion  OutDataTypeStr=int32  RndMeth=Nearest  SaturateOnIntegerOverflow=off
  Data Type Conversion7 : DataTypeConversion  OutDataTypeStr=single  RndMeth=Nearest  SaturateOnIntegerOverflow=off
  Divide : Product  Inputs=*/
  Gain1 : Gain  Gain=0.25  SaturateOnIntegerOverflow=on  OutDataTypeStr=Inherit: Same as input  ParamDataTypeStr=Inherit: Same as input
  Gain2 : Gain  Gain=-1  SaturateOnIntegerOverflow=on  OutDataTypeStr=Inherit: Same as input  ParamDataTypeStr=Inherit: Same as input
  Relational Operator1 : RelationalOperator
  Relational Operator2 : RelationalOperator  Operator=<
  Set-Reset Flip-Flop : eeGeneralControl/Set-Reset Flip-Flop  LabelModeActiveChoice=Discrete  UndefState=Set  Q0=0  Ts=Ts
      settings: LibrarySourceBlock=ee_sl_lib/General Control/Set-Reset Flip-Flop
  Sum2 : Sum  InputSameDT=on  SaturateOnIntegerOverflow=on  OutDataTypeStr=Inherit: Same as first input
  Switch : Switch  Criteria=u2 ~= 0
  Unit Delay1 : UnitDelay  SampleTime=Ts  HasFrameUpgradeWarning=on
  Unit Delay2 : UnitDelay  SampleTime=Ts  HasFrameUpgradeWarning=on
  Triangle : Outport  InitialOutput=0  VectorParamsAs1DForOutWhenUnconnected=off
  wires:
  Constat/1 -> Switch/1
  Constat1/1 -> Switch/3
  Switch/1 -> Sum2/1
  Unit Delay1/1 -> Sum2/2
  Sum2/1 -> Relational Operator2/1, Relational Operator1/1, Unit Delay1/1, Data Type Conversion7/1
  Gain1/1 -> Divide/2, Data Type Conversion1/1
  Relational Operator1/1 -> Set-Reset Flip-Flop/1
  Gain2/1 -> Relational Operator2/2
  Relational Operator2/1 -> Set-Reset Flip-Flop/2
  Set-Reset Flip-Flop/1 -> Unit Delay2/1
  Unit Delay2/1 -> Switch/2
  Divide/1 -> Triangle/1
  Data Type Conversion7/1 -> Divide/1  "Simulink-PS Converter1"
  steps/1 -> Gain1/1  "Simulink-PS Converter1"
  Data Type Conversion1/1 -> Gain2/1, Relational Operator1/2  "Simulink-PS Converter1"

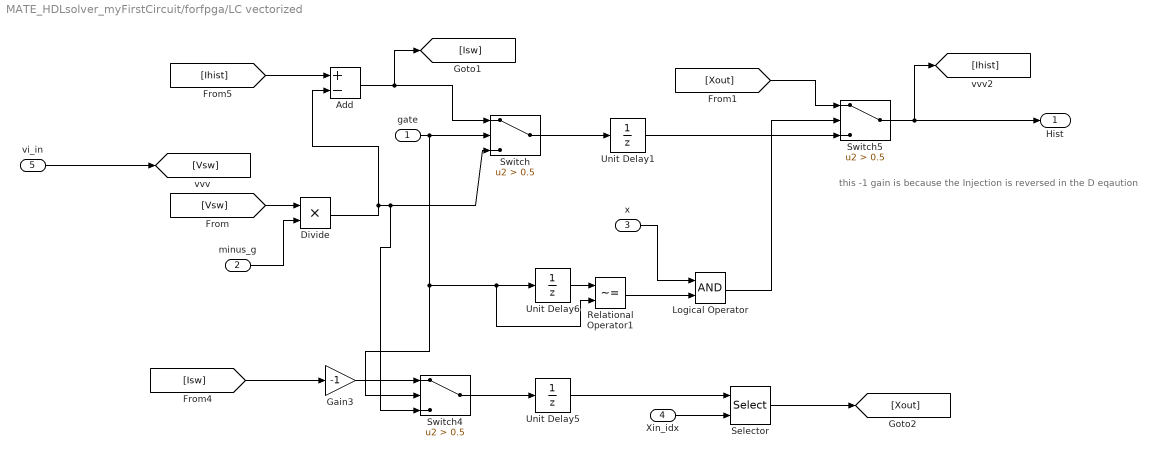
== system MATE_HDLsolver_myFirstCircuit/forfpga/LC vectorized ==
  note: this -1 gain is because the Injection is reversed in the D eqaution
  gate : Inport
  minus_g : Inport  Port=2
  x : Inport  Port=3
  Xin_idx : Inport  Port=4
  vi_in : Inport  Port=5
  Add : Sum  Inputs=+-
  Divide : Product
  Gain3 : Gain  Gain=-1
  Logical Operator : Logic  AllPortsSameDT=off  OutDataTypeStr=boolean
  Relational Operator1 : RelationalOperator  Operator=~=  OutDataTypeStr=boolean  RndMeth=Simplest  InputSameDT=off
  Selector : Selector  InputPortWidth=5  IndexOptions=Index vector (port)  Indices=[2 1 3 4 5]  OutputSizes=1
  Switch : Switch  Criteria=u2 > Threshold  Threshold=0.5  SaturateOnIntegerOverflow=off  InputSameDT=off
  Switch4 : Switch  Criteria=u2 > Threshold  Threshold=0.5  SaturateOnIntegerOverflow=off  InputSameDT=off
  Switch5 : Switch  Criteria=u2 > Threshold  Threshold=0.5  SaturateOnIntegerOverflow=off  InputSameDT=off
  Unit Delay1 : UnitDelay  SampleTime=Ts  HasFrameUpgradeWarning=on
  Unit Delay5 : UnitDelay  SampleTime=Ts  HasFrameUpgradeWarning=on
  Unit Delay6 : UnitDelay  SampleTime=Ts  HasFrameUpgradeWarning=on
  Hist : Outport
  wires:
  [Vsw] -> Divide/1
  [Ihist] -> Add/1
  Add/1 -> [Isw], Switch/1
  Switch/1 -> Unit Delay1/1
  vi_in/1 -> [Vsw]
  Unit Delay1/1 -> Switch5/3
  minus_g/1 -> Divide/2
  Switch5/1 -> Hist/1, [Ihist]
  Divide/1 -> Switch4/3, Switch/3, Add/2
  Switch4/1 -> Unit Delay5/1
  Unit Delay5/1 -> Selector/1
  gate/1 -> Switch/2, Switch4/2, Relational Operator1/2, Unit Delay6/1
  [Isw] -> Gain3/1
  Gain3/1 -> Switch4/1
  Unit Delay6/1 -> Relational Operator1/1
  [Xout] -> Switch5/1
  Relational Operator1/1 -> Logical Operator/2
  Logical Operator/1 -> Switch5/2
  x/1 -> Logical Operator/1
  Selector/1 -> [Xout]
  Xin_idx/1 -> Selector/2

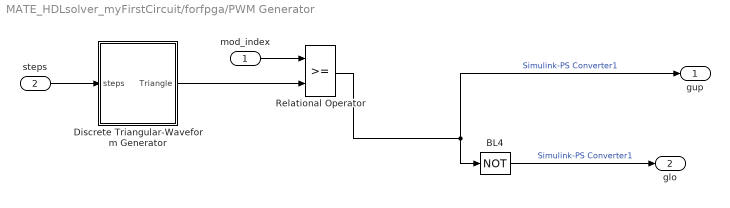
== system MATE_HDLsolver_myFirstCircuit/forfpga/PWM Generator ==
  mod_index : Inport
  steps : Inport  Port=2
  BL4 : Logic  Operator=NOT  Inputs=1
  Discrete Triangular-Waveform Generator : Subsystem
  Relational Operator : RelationalOperator  OutDataTypeStr=boolean
  gup : Outport  VectorParamsAs1DForOutWhenUnconnected=off
  glo : Outport  Port=2  VectorParamsAs1DForOutWhenUnconnected=off
  wires:
  Discrete Triangular-Waveform Generator/1(Triangle) -> Relational Operator/2
  mod_index/1 -> Relational Operator/1
  steps/1 -> Discrete Triangular-Waveform Generator/1(steps)
  Relational Operator/1 -> gup/1, BL4/1  "Simulink-PS Converter1"
  BL4/1 -> glo/1  "Simulink-PS Converter1"

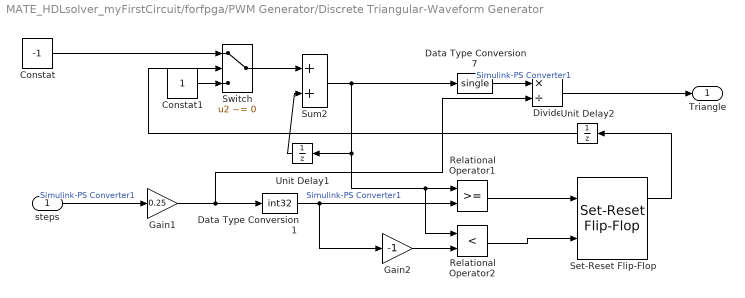
== system MATE_HDLsolver_myFirstCircuit/forfpga/PWM Generator/Discrete Triangular-Waveform Generator ==
  steps : Inport
  Constat : Constant  Value=-1  OutDataTypeStr=int32
  Constat1 : Constant  OutDataTypeStr=int32
  Data Type Conversion1 : DataTypeConversion  OutDataTypeStr=int32  RndMeth=Nearest  SaturateOnIntegerOverflow=off
  Data Type Conversion7 : DataTypeConversion  OutDataTypeStr=single  RndMeth=Nearest  SaturateOnIntegerOverflow=off
  Divide : Product  Inputs=*/
  Gain1 : Gain  Gain=0.25  SaturateOnIntegerOverflow=on  OutDataTypeStr=Inherit: Same as input  ParamDataTypeStr=Inherit: Same as input
  Gain2 : Gain  Gain=-1  SaturateOnIntegerOverflow=on  OutDataTypeStr=Inherit: Same as input  ParamDataTypeStr=Inherit: Same as input
  Relational Operator1 : RelationalOperator
  Relational Operator2 : RelationalOperator  Operator=<
  Set-Reset Flip-Flop : eeGeneralControl/Set-Reset Flip-Flop  LabelModeActiveChoice=Discrete  UndefState=Set  Q0=0  Ts=Ts
      settings: LibrarySourceBlock=ee_sl_lib/General Control/Set-Reset Flip-Flop
  Sum2 : Sum  InputSameDT=on  SaturateOnIntegerOverflow=on  OutDataTypeStr=Inherit: Same as first input
  Switch : Switch  Criteria=u2 ~= 0
  Unit Delay1 : UnitDelay  SampleTime=Ts  HasFrameUpgradeWarning=on
  Unit Delay2 : UnitDelay  SampleTime=Ts  HasFrameUpgradeWarning=on
  Triangle : Outport  InitialOutput=0  VectorParamsAs1DForOutWhenUnconnected=off
  wires:
  Constat/1 -> Switch/1
  Constat1/1 -> Switch/3
  Switch/1 -> Sum2/1
  Unit Delay1/1 -> Sum2/2
  Sum2/1 -> Relational Operator2/1, Relational Operator1/1, Unit Delay1/1, Data Type Conversion7/1
  Gain1/1 -> Divide/2, Data Type Conversion1/1
  Relational Operator1/1 -> Set-Reset Flip-Flop/1
  Gain2/1 -> Relational Operator2/2
  Relational Operator2/1 -> Set-Reset Flip-Flop/2
  Set-Reset Flip-Flop/1 -> Unit Delay2/1
  Unit Delay2/1 -> Switch/2
  Divide/1 -> Triangle/1
  Data Type Conversion7/1 -> Divide/1  "Simulink-PS Converter1"
  steps/1 -> Gain1/1  "Simulink-PS Converter1"
  Data Type Conversion1/1 -> Gain2/1, Relational Operator1/2  "Simulink-PS Converter1"
